simulink model "vhs_fpga_tx_10k_nosmq_nodsp"  (Simulink 7.1)
settings: Solver=ode45  StartTime=0.0  StopTime=inf  RelTol=1e-3
PreLoadFcn:
  | parameter();
undefined symbols (not defined in the file or in its folder): N1_CIC_PRESET1, N_FB_RX_frame, N_FB_TX_frame
libraries: xbsIndex_r4 x95, vhsadac_common_ob_fpgalib_v1_2_0 x10, misc_tools_dsplib_v1_0_0 x1, misc_tools_fpgalib_v1_0_0 x1, rffe_fpgalib_v1_1_0 x1, rtdex_fpgalib_v1_1_0 x1
(part 1 of 2)
settings Model: Creator=comlab  LastModifiedBy=lyrtech

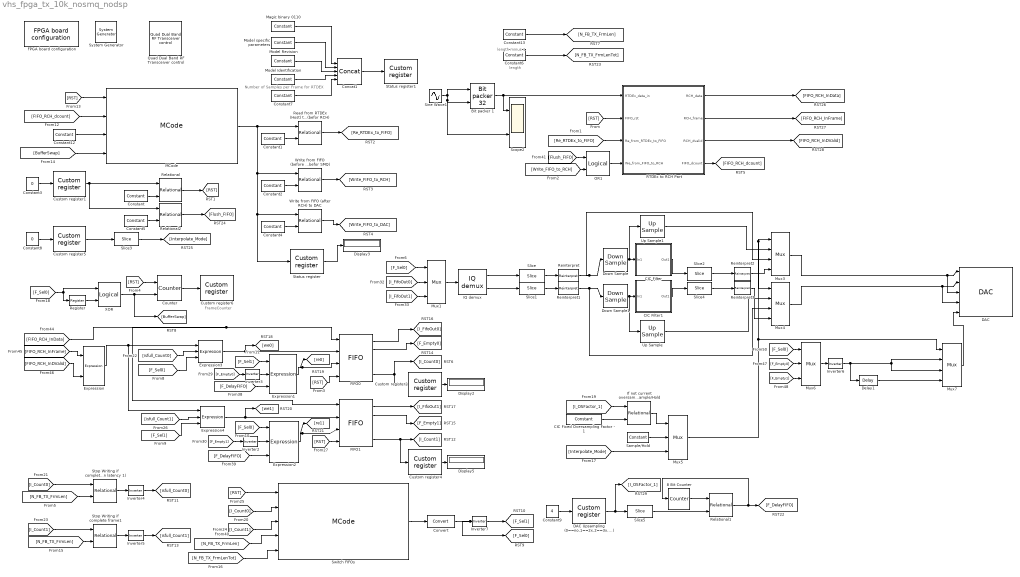
== system vhs_fpga_tx_10k_nosmq_nodsp ==
  note: FrameCounter
  note: length minus 1
  note: length
  note: Number of Samples per Frame for RTDEX
  " System Generator" : xbsIndex_r4/ System Generator  Tag=genX  SystemSampleTime=-1  xilinxfamily=virtex4  part=xc4vsx55  speed=-10  package=ff1148  synthesis_tool=XST  clock_wrapper=Clock Enables  directory=./netlist  testbench=off  simulink_period=1  sysclk_period=9  dcm_input_clock_period=100  incr_netlist=off  trim_vbits=Everywhere in SubSystem  dbl_ovrd=According to Block Masks  core_generation=According to Block Masks  run_coregen=off  deprecated_control=off  eval_field=0  block_type=sysgen
      settings: block_version=10.1.3
  8 Bit Counter : xbsIndex_r4/Counter  cnt_type=Free Running  cnt_to=Inf  operation=Up  start_count=0  cnt_by_val=1  arith_type=Unsigned  n_bits=8  bin_pt=0  load_pin=off  rst=on  en=off  explicit_period=on  period=1  dbl_ovrd=off  use_behavioral_HDL=off  use_rpm=off  implementation=Fabric  block_type=counter
      settings: block_version=VER_STRING_GOES_HERE
  Bit packer 1 : misc_tools_dsplib_v1_0_0/Bit packer 32  Tag=LYR_DSP_MISC_BIT_PACKER_32  Description=Lyrtech block  input_descriptor=[-16 -16]  data_type=double  frame_size=1
  CIC Filter : Subsystem  mask(CIC Filter){input_bitwidth=14, input_binpt=0, filter_type=Interpolator, rate_change=N1_CIC_PRESET1, stages=3, m=1, pipeline=on}
      mask prompts: input_bitwidth "Input Bit Width"; input_binpt "Input Binary Point"; filter_type "Filter Type"; rate_change "Sample Rate Change"; stages "Number of Stages"; m "Differential Delay"; pipeline "Pipeline Differentiators"
      mask help: Cascaded Integrated Comb (CIC) Filter
      mask init:
      | % CIC Single Channel v1.0
      | % Set Block Logo
      | sav_gcb=gcb;
      | [bg,fg] = xlcmap('XBlock',0);
      | iPos = get_param(sav_gcb,'Position');
      | iWidth=iPos(3)-iPos(1); iHeight=iPos(4)-iPos(2);
      | iCx=iWidth/2;
      | iCy=iHeight/2;
      | [logoX, logoY] = xlogo(iPos);
      | 
      | % Determine previous filter type and number of stages
      | prev_stages_list = find_system(sav_gcb, 'lookUnderMasks', 'all', 'FollowLinks', 'on', 'Regexp', 'on', 'Name', '^Integrator*'); %this is a cell array
      | prev_stages = length(prev_stages_list);
      | 
      | prev_filter_list = find_system(sav_gcb, 'lookUnderMasks', 'all', 'FollowLinks', 'on', 'Regexp', 'on', 'Name', '^Up Sample*'); %this is a cell array
      | if (isempty(prev_filter_list))
      |     prev_filter_list = find_system(sav_gcb, 'lookUnderMasks', 'all', 'FollowLinks', 'on', 'Regexp', 'on', 'Name', '^Down Sample*'); %this is a cell array
      |     if (isempty(prev_filter_list))
      |         errordlg('Previous Filter Type could not be determined')
      |     else
      |         prev_filter_type = 2;
      |     end
      | else
      |     prev_filter_type = 1;
      | end
      |   
      |   
      | % Print label on the block
      | if(filter_type == 2)
      |    cic_str = sprintf('%d-Stage\n CIC\n%d:1 Decimator',stages, rate_change);
      | else
      |    cic_str = sprintf('%d-Stage\n CIC\n1:%d Interpolator',stages, rate_change);	
      | end
      | 
      | % Make sure the entered values for stages and channels are positive integers
      | nstages = round(sum(abs(stages)));
      | 
      | % issue an error if the number of stages entered is zero
      | if (nstages == 0)
      | 	nstages = prev_stages;
      | 	errordlg('Number of Stages must be more than zero')
      | end
      | 
      | if (nstages == prev_stages) & (filter_type == prev_filter_type)
      |     return
      | end
      | 
      | if(filter_type == 2) % Decimator
      |    if (prev_filter_type == 1) % was interpolator so turn to decimator
      |        for i= 2:prev_stages,
      | 	      delete_line(sav_gcb, ['Integrator' int2str(i-1) '/' int2str(1)], ['Integrator' int2str(i) '/' int2str(1)]);
      | 	      delete_line(sav_gcb, ['Differentiator' int2str(i-1) '/' int2str(1)], ['Differentiator' int2str(i) '/' int2str(1)]);
      |        end
      | 
      |        % disconnect the last blocks in the two sections
      |        delete_line(sav_gcb, ['Differentiator' int2str(prev_stages) '/' int2str(1)], ['Up Sample/1']);
      |        delete_line(sav_gcb, ['Integrator' int2str(prev_stages) '/' int2str(1)], 'Out1/1');
      | 	
      | 	   % delete the line from the Up sampler to the Integrator
      | 	   delete_line(sav_gcb, 'Up Sample/1', 'Integrator1/1'); 
      | 	   delete_line(sav_gcb, 'In1/1', 'Differentiator1/1'); 
      | 	   
      | 	   % Delete the Up Sampler and then replace with an Down Sampler
      | 	   pup = get_param([sav_gcb '/Up Sample'], 'position');
      | 	   delete_block([sav_gcb '/Up Sample']);
      | 	   load_system('xbsIndex_r4');
      | 	   add_block('xbsIndex_r4/Down Sample', [sav_gcb '/Down Sample'], 'sample_ratio', 'rate_change','sample_phase', 'First Value of Frame', 'position', [pup(1), pup(2), pup(3),pup(4)]);
      | 	   
      | 	   % Switch the Integrators and Decimators around
      | 	   for i=1:prev_stages,
      | 		   tempi = get_param([sav_gcb '/Integrator' int2str(i)], 'position');
      | 	       tempd = get_param([sav_gcb '/Differentiator' int2str(i)], 'position');
      | 		   set_param([sav_gcb '/Differentiator' int2str(i)], 'position', [tempi(1), tempi(2), tempi(3), tempi(4)], 'output_bitwidth', 'ceil(stages*log2(rate_change*m) + input_bitwidth)');
      | 		   set_param([sav_gcb '/Integrator' int2str(i)], 'position', [tempd(1), tempd(2), tempd(3), tempd(4)]);
      | 	   end
      | 	   	   	
      | 	   % add back in the lines
      |        add_line(sav_gcb, 'In1/1', 'Integrator1/1', 'autorouting', 'on');
      | 	   add_line(sav_gcb, ['Integrator' int2str(prev_stages) '/1'], 'Down Sample/1', 'autorouting', 'on');
      | 	   add_line(sav_gcb, 'Down Sample/1', 'Differentiator1/1', 'autorouting', 'on');
      | 	   add_line(sav_gcb, ['Differentiator' int2str(prev_stages) '/1'], 'Out1/1', 'autorouting', 'on');
      | 	   for i= 2:prev_stages,
      |           add_line(sav_gcb, ['Integrator' int2str(i-1) '/1'], ['Integrator' int2str(i) '/' int2str(1)], 'autorouting', 'on');
      |           add_line(sav_gcb, ['Differentiator' int2str(i-1) '/1'], ['Differentiator' int2str(i) '/' int2str(1)], 'autorouting', 'on');
      | 	   end
      | 		
      |        %Set the Output bit widths of Differentiator and Integrator stages
      |        set_param([sav_gcb '/Differentiator1'], 'output_bitwidth', 'ceil(stages*log2(rate_change*m) + input_bitwidth)');
      | 	   	   %Set the Output bit width of Integrator stages
      | 	   %Calculate the Interpolator Integrator Output Bit Growth
      |        for i= 1:prev_stages,
      | 			 j = nstages+i;
      | 	         set_param([sav_gcb '/Integrator' int2str(i)], 'output_bitwidth', 'ceil(stages*log2(rate_change*m) + input_bitwidth)');
      |              set_param([sav_gcb '/Differentiator' int2str(i)], 'output_bitwidth', 'ceil(stages*log2(rate_change*m) + input_bitwidth)');
      | 	   end
      | 	   
      |    end
      |    
      |    if (nstages ~= prev_stages)
      |     
      |        % disconnect all the wires from all the blocks
      |        for i= 2:prev_stages,
      | 	      delete_line(sav_gcb, ['Integrator' int2str(i-1) '/' int2str(1)], ['Integrator' int2str(i) '/' int2str(1)]);
      | 	      delete_line(sav_gcb, ['Differentiator' int2str(i-1) '/' int2str(1)], ['Differentiator' int2str(i) '/' int2str(1)]);
      |        end
      | 
      |        % disconnect the last blocks in the two sections
      |        delete_line(sav_gcb, ['Integrator' int2str(prev_stages) '/' int2str(1)], ['Down Sample/1']);
      |        delete_line(sav_gcb, ['Differentiator' int2str(prev_stages) '/' int2str(1)], 'Out1/1');
      | 	
      | 	   % delete the line from the down sampler to the differentiator
      | 	   delete_line(sav_gcb, 'Down Sample/1', 'Differentiator1/1');
      | 	
      | 	   % Remove all the blocks except the first one (as we always will have one)
      |        for i=2:prev_stages,
      | 		  delete_block([sav_gcb '/Differentiator' int2str(i)]);
      | 	      delete_block([sav_gcb '/Integrator' int2str(i)]);
      |        end
      | 	   
      | 	   %Set the Output bit width of Differentiator stages
      |        set_param([sav_gcb '/Differentiator1'], 'output_bitwidth', 'ceil(stages*log2(rate_change*m) + input_bitwidth)');
      | 	   
      | 	   % collect data on the position of existing blocks
      | 	   pi = get_param([sav_gcb '/Integrator1'], 'position');
      | 	   pd = get_param([sav_gcb '/Differentiator1'], 'position');
      | 	   set_param([sav_gcb '/Differentiator1'], 'position', [pi(1)+(nstages+1)*80, pd(2), pi(3)+(nstages+1)*80, pd(4)]);
      | 	   pd = get_param([sav_gcb '/Differentiator1'], 'position');
      | 	
      | 	   % move the current blocks to accomadate for new blocks to be added 
      | 	   pds = get_param([sav_gcb '/Down Sample'], 'position');
      | 	   set_param([sav_gcb '/Down Sample'], 'position', [pi(1)+(nstages)*80, pds(2), pi(3)+(nstages)*80, pds(4)]);
      | 	   
      | 	   po = get_param([sav_gcb '/Out1'], 'position');
      | 	   set_param([sav_gcb '/Out1'], 'position', [pd(1)+(nstages+1)*80, po(2), pd(1)+(po(3)-po(1))+(nstages+1)*80, po(4)]);	
      | 	
      | 	   % add back in the line between the Down Sampler and the 1st Differentiator
      |        add_line(sav_gcb, 'Down Sample/1', ['Differentiator1/' int2str(1)], 'autorouting', 'on');
      | 
      | 	   % Only add blocks if more than one stage is required
      | 	   if (nstages ~= 1)
      | 		
      | 	       % Add in a copy of the first block to make up the required number of stages
      |            for i=2:nstages,
      |                add_block([sav_gcb '/Integrator1'], [sav_gcb '/Integrator' int2str(i)], 'position', [pi(1)+(i-1)*80, pi(2), pi(3)+(i-1)*80, pi(4)]);
      | 		       add_block([sav_gcb '/Differentiator1'], [sav_gcb '/Differentiator' int2str(i)], 'position', [pd(1)+(i-1)*80, pd(2), pd(3)+(i-1)*80, pd(4)]);
      | 	       end
      | 		
      | 	       % Connect up the wires to each block use autorouting
      |            for i= 2:nstages,
      |  		       add_line(sav_gcb, ['Integrator' int2str(i-1) '/' int2str(1)], ['Integrator' int2str(i) '/' int2str(1)], 'autorouting', 'on');
      | 	           add_line(sav_gcb, ['Differentiator' int2str(i-1) '/' int2str(1)], ['Differentiator' int2str(i) '/' int2str(1)], 'autorouting', 'on');
      |            end
      | 	    end
      | 	       % Connect the last blocks in the two sections
      |            add_line(sav_gcb, ['Integrator' int2str(nstages) '/' int2str(1)], ['Down Sample/1'], 'autorouting', 'on');
      |            add_line(sav_gcb, ['Differentiator' int2str(nstages) '/' int2str(1)], ['Out1/1'], 'autorouting', 'on');
      |    end
      | 
      | else % Interpolator
      |    
      | 	
      | 	if (prev_filter_type == 2) % was decimator so turn to interpolator
      | 	
      | 	  % disconnect all the wires from all the blocks
      |        for i= 2:prev_stages,
      | 	      delete_line(sav_gcb, ['Integrator' int2str(i-1) '/' int2str(1)], ['Integrator' int2str(i) '/' int2str(1)]);
      | 	      delete_line(sav_gcb, ['Differentiator' int2str(i-1) '/' int2str(1)], ['Differentiator' int2str(i) '/' int2str(1)]);
      |        end
      | 
      |        % disconnect the last blocks in the two sections
      |        delete_line(sav_gcb, ['Integrator' int2str(prev_stages) '/' int2str(1)], ['Down Sample/1']);
      |        delete_line(sav_gcb, ['Differentiator' int2str(prev_stages) '/' int2str(1)], 'Out1/1');
      | 	
      | 	   % delete the line from the down sampler to the Differentiator
      | 	   delete_line(sav_gcb, 'Down Sample/1', 'Differentiator1/1'); 
      | 	   delete_line(sav_gcb, 'In1/1', 'Integrator1/1'); 
      | 	   
      | 	   % Delete the Down Sampler and then replace with a Up Sampler
      | 	   pdwn = get_param([sav_gcb '/Down Sample'], 'position');
      | 	   delete_block([sav_gcb '/Down Sample']);
      | 	   load_system('xbsIndex_r4');
      | 	   add_block('xbsIndex_r4/Up Sample', [sav_gcb '/Up Sample'], 'sample_ratio', 'rate_change', 'position', [pdwn(1), pdwn(2), pdwn(3), pdwn(4)]);
      | 	   
      | 	   % Switch the Integrators and Decimators around
      | 	   for i=1:prev_stages,
      | 		   tempi = get_param([sav_gcb '/Integrator' int2str(i)], 'position');
      | 	       tempd = get_param([sav_gcb '/Differentiator' int2str(i)], 'position');
      | 		   set_param([sav_gcb '/Differentiator' int2str(i)], 'position', [tempi(1), tempi(2), tempi(3), tempi(4)], 'output_bitwidth', [int2str(i) '+ input_bitwidth']);
      | 		   set_param([sav_gcb '/Integrator' int2str(i)], 'position', [tempd(1), tempd(2), tempd(3), tempd(4)]);
      | 	   end
      | 	   	   	
      | 	   % add back in the lines
      |        add_line(sav_gcb, 'In1/1', 'Differentiator1/1', 'autorouting', 'on');
      | 	   add_line(sav_gcb, ['Differentiator' int2str(prev_stages) '/1'], 'Up Sample/1', 'autorouting', 'on');
      | 	   add_line(sav_gcb, 'Up Sample/1', 'Integrator1/1', 'autorouting', 'on');
      | 	   add_line(sav_gcb, ['Integrator' int2str(prev_stages) '/1'], 'Out1/1', 'autorouting', 'on');
      | 	   for i= 2:prev_stages,
      |           add_line(sav_gcb, ['Integrator' int2str(i-1) '/1'], ['Integrator' int2str(i) '/1'], 'autorouting', 'on');
      |           add_line(sav_gcb, ['Differentiator' int2str(i-1) '/1'], ['Differentiator' int2str(i) '/1'], 'autorouting', 'on');
      | 	   end
      | 	   
      | 	   %Set the Output bit width of Integrator stages
      | 	   %Calculate the Interpolator Integrator Output Bit Growth
      |        for i= 1:prev_stages,
      | 			 j = nstages+i;
      | 	         set_param([sav_gcb '/Integrator' int2str(i)], 'output_bitwidth', ['ceil(log2(2^(2*stages-' int2str(j) ')*(rate_change*m)^(' int2str(j) '-stages)) + input_bitwidth)']);
      | 	   end
      | 		
      |    end
      |    
      | 	
      | 	if (nstages ~= prev_stages)
      |     
      |        % disconnect all the wires from all the blocks
      |        for i= 2:prev_stages,
      | 	      delete_line(sav_gcb, ['Integrator' int2str(i-1) '/' int2str(1)], ['Integrator' int2str(i) '/' int2str(1)]);
      | 	      delete_line(sav_gcb, ['Differentiator' int2str(i-1) '/' int2str(1)], ['Differentiator' int2str(i) '/' int2str(1)]);
      |        end
      | 
      |        % disconnect the last blocks in the two sections
      |        delete_line(sav_gcb, ['Differentiator' int2str(prev_stages) '/' int2str(1)], ['Up Sample/1']);
      |        delete_line(sav_gcb, ['Integrator' int2str(prev_stages) '/' int2str(1)], 'Out1/1');
      |        
      | 	
      | 	   % delete the line from the Up sampler to the Integrator1 for movement later
      | 	   delete_line(sav_gcb, 'Up Sample/1', 'Integrator1/1'); 
      | 	
      | 	   % Remove all the blocks except the first one (as we always will have one)
      |        for i=2:prev_stages,
      | 		  delete_block([sav_gcb '/Differentiator' int2str(i)]);
      | 	      delete_block([sav_gcb '/Integrator' int2str(i)]);
      |        end
      | 	
      | 	   %Set the Output bit width of first Differentiator stage (other are set as copies of this block)
      |        set_param([sav_gcb '/Differentiator1'], 'output_bitwidth', '1 + input_bitwidth');
      | 	   
      | 	   % collect data on the position of existing blocks
      | 	   pi = get_param([sav_gcb '/Integrator1'], 'position');
      | 	   pd = get_param([sav_gcb '/Differentiator1'], 'position');
      | 	   set_param([sav_gcb '/Integrator1'], 'position', [pd(1)+(nstages+1)*80, pi(2), pd(3)+(nstages+1)*80, pi(4)]);
      | 	   pi = get_param([sav_gcb '/Integrator1'], 'position');
      | 	
      | 	   % move the current blocks to accomadate for new blocks to be added 
      | 	   pus = get_param([sav_gcb '/Up Sample'], 'position');
      | 	   set_param([sav_gcb '/Up Sample'], 'position', [pd(1)+(nstages)*80, pus(2), pd(3)+(nstages)*80, pus(4)]);
      | 	
      | 	   po = get_param([sav_gcb '/Out1'], 'position');
      |        set_param([sav_gcb '/Out1'], 'position', [pi(1)+(nstages+1)*80, po(2), pi(1)+(po(3)-po(1))+(nstages+1)*80, po(4)]);	
      |       
      | 	
      | 	   % add back in the line between the Up Sampler and the 1st Integrator1
      | 	   add_line(sav_gcb, 'Up Sample/1', 'Integrator1/1', 'autorouting', 'on');
      | 	   
      | 	   % Only add blocks if more than one stage is required
      | 	   if (nstages ~= 1)
      | 		
      | 	       % Add in a copy of the first block to make up the required number of stages
      |            for i=2:nstages,
      |                add_block([sav_gcb '/Integrator1'], [sav_gcb '/Integrator' int2str(i)], 'position', [pi(1)+(i-1)*80, pi(2), pi(3)+(i-1)*80, pi(4)]);
      | 		       add_block([sav_gcb '/Differentiator1'], [sav_gcb '/Differentiator' int2str(i)], 'position', [pd(1)+(i-1)*80, pd(2), pd(3)+(i-1)*80, pd(4)], 'output_bitwidth', [int2str(i) '+ input_bitwidth']);
      | 	       end
      | 		
      | 	       % Connect up the wires to each block use autorouting
      |            for i= 2:nstages,
      |  		       add_line(sav_gcb, ['Integrator' int2str(i-1) '/' int2str(1)], ['Integrator' int2str(i) '/' int2str(1)], 'autorouting', 'on');
      | 	           add_line(sav_gcb, ['Differentiator' int2str(i-1) '/' int2str(1)], ['Differentiator' int2str(i) '/' int2str(1)], 'autorouting', 'on');
      |            end
      | 	    end
      | 	       % Connect the last blocks in the two sections
      |            add_line(sav_gcb, ['Differentiator' int2str(nstages) '/1'], ['Up Sample/1'], 'autorouting', 'on');
      |            add_line(sav_gcb, ['Integrator' int2str(nstages) '/1'], ['Out1/1'], 'autorouting', 'on');
      | 		   
      | 	     %Set the Output bit width of Integrator stages
      | 	     %Calculate the Interpolator Integrator Output Bit Growth
      |           for i= 1:nstages,
      | 			 j = nstages+i;
      | 	         set_param([sav_gcb '/Integrator' int2str(i)], 'output_bitwidth', ['ceil(log2(2^(2*stages-' int2str(j) ')*(rate_change*m)^(' int2str(j) '-stages)) + input_bitwidth)']);
      | 	      end
      |    end
      | 	  
      | end
      | 
      | 
      | % Set the pipelining to ON or OFF on the differentiators
      | if (pipeline == 0)
      | 	for i= 1:nstages
      | 		set_param([sav_gcb '/Differentiator' int2str(i), '/AddSub'], 'latency', '0')
      | 	end
      | else
      | 	for i= 1:nstages
      | 		set_param([sav_gcb '/Differentiator' int2str(i), '/AddSub'], 'latency' ,'1')
      | 	end
      | end
      settings: CopyFcn=set_param(gcb, 'MaskSelfModifiable', 'on', 'LinkStatus', 'none');
      mask Help: eval('');xlDoc('-book','sysgen','-topic','CIC_Filter');
      mask StyleString: edit,edit,popup(Interpolator|Decimator),edit,edit,popup(1|2|3|4),checkbox
      mask Display:
      | patch([0 iWidth iWidth 0],[0 0 iHeight iHeight] , bg);
      | patch(logoX,logoY , fg);
      | plot([0 0 iWidth iWidth 0], [0 iHeight iHeight 0 0]);
      | disp(cic_str)
  CIC Filter1 : Subsystem  mask(CIC Filter){input_bitwidth=14, input_binpt=0, filter_type=Interpolator, rate_change=N1_CIC_PRESET1, stages=3, m=1, pipeline=on}
      mask prompts: input_bitwidth "Input Bit Width"; input_binpt "Input Binary Point"; filter_type "Filter Type"; rate_change "Sample Rate Change"; stages "Number of Stages"; m "Differential Delay"; pipeline "Pipeline Differentiators"
      mask help: Cascaded Integrated Comb (CIC) Filter
      mask init: same as vhs_fpga_tx_10k_nosmq_nodsp/CIC Filter
      settings: CopyFcn=set_param(gcb, 'MaskSelfModifiable', 'on', 'LinkStatus', 'none');
      mask Help: eval('');xlDoc('-book','sysgen','-topic','CIC_Filter');
      mask StyleString: edit,edit,popup(Interpolator|Decimator),edit,edit,popup(1|2|3|4),checkbox
      mask Display:
      | patch([0 iWidth iWidth 0],[0 0 iHeight iHeight] , bg);
      | patch(logoX,logoY , fg);
      | plot([0 0 iWidth iWidth 0], [0 iHeight iHeight 0 0]);
      | disp(cic_str)
  CIC Fixed Oversampling Factor - 1 : xbsIndex_r4/Constant  arith_type=Unsigned  const=N1_CIC_PRESET1-1  n_bits=32  bin_pt=0  explicit_period=on  period=1  equ=P=C  opselect=C  inp2=PCIN>>17  opr=+  inp1=P  carry=CIN  dbl_ovrd=off  block_type=constant
  Concat1 : xbsIndex_r4/Concat  num_inputs=5  dbl_ovrd=off  block_type=concat
      settings: block_version=10.1.3
  Constant : xbsIndex_r4/Constant  arith_type=Unsigned  const=1  n_bits=32  bin_pt=0  explicit_period=off  period=1  equ=P=C  opselect=C  inp2=PCIN>>17  opr=+  inp1=P  carry=CIN  dbl_ovrd=off  block_type=constant
  Constant1 : xbsIndex_r4/Constant  arith_type=Unsigned  const=1  n_bits=32  bin_pt=0  explicit_period=on  period=1  equ=P=C  opselect=C  inp2=PCIN>>17  opr=+  inp1=P  carry=CIN  dbl_ovrd=off  block_type=constant
  Constant12 : xbsIndex_r4/Constant  arith_type=Unsigned  const=N_FB_RX_frame  n_bits=14  bin_pt=0  explicit_period=on  period=1  equ=P=C  opselect=C  inp2=PCIN>>17  opr=+  inp1=P  carry=CIN  dbl_ovrd=off  block_type=constant
  Constant13 : xbsIndex_r4/Constant  arith_type=Unsigned  const=N_FB_TX_frame-1  n_bits=14  bin_pt=0  explicit_period=on  period=1  equ=P=C  opselect=C  inp2=PCIN>>17  opr=+  inp1=P  carry=CIN  dbl_ovrd=off  block_type=constant
  Constant2 : xbsIndex_r4/Constant  arith_type=Unsigned  const=2  n_bits=32  bin_pt=0  explicit_period=on  period=1  equ=P=C  opselect=C  inp2=PCIN>>17  opr=+  inp1=P  carry=CIN  dbl_ovrd=off  block_type=constant
  Constant3 : Constant  Value=0  OutDataType=sfix(16)  OutScaling=2^0  SampleTime=1
  Constant4 : xbsIndex_r4/Constant  arith_type=Unsigned  const=3  n_bits=32  bin_pt=0  explicit_period=on  period=1  equ=P=C  opselect=C  inp2=PCIN>>17  opr=+  inp1=P  carry=CIN  dbl_ovrd=off  block_type=constant
  Constant5 : xbsIndex_r4/Constant  arith_type=Unsigned  const=2  n_bits=32  bin_pt=0  explicit_period=off  period=1  equ=P=C  opselect=C  inp2=PCIN>>17  opr=+  inp1=P  carry=CIN  dbl_ovrd=off  block_type=constant
  Constant6 : xbsIndex_r4/Constant  arith_type=Unsigned  const=N_FB_TX_frame  n_bits=14  bin_pt=0  explicit_period=on  period=1  equ=P=C  opselect=C  inp2=PCIN>>17  opr=+  inp1=P  carry=CIN  dbl_ovrd=off  block_type=constant
  Constant7 : xbsIndex_r4/Constant  arith_type=Unsigned  const=N_FB_RX_frame  n_bits=15  bin_pt=0  explicit_period=on  period=1  equ=P=C  opselect=C  inp2=PCIN>>17  opr=+  inp1=P  carry=CIN  dbl_ovrd=off  block_type=constant
  Constant8 : Constant  Value=0  OutDataType=sfix(16)  OutScaling=2^0  SampleTime=1
  Constant9 : Constant  Value=4  OutDataType=sfix(16)  OutScaling=2^0  SampleTime=1
  Convert : xbsIndex_r4/Convert  arith_type=Boolean  n_bits=1  bin_pt=0  quantization=Truncate  overflow=Wrap  latency=2  dbl_ovrd=off  pipeline=off  block_type=convert
      settings: block_version=10.1.3
  Counter : xbsIndex_r4/Counter  cnt_type=Free Running  cnt_to=Inf  operation=Up  start_count=0  cnt_by_val=1  arith_type=Unsigned  n_bits=32  bin_pt=0  load_pin=off  rst=on  en=on  explicit_period=on  period=1  dbl_ovrd=off  use_behavioral_HDL=off  use_rpm=off  implementation=Fabric  block_type=counter
  Custom register1 : vhsadac_common_ob_fpgalib_v1_2_0/Custom register  Tag=LYR_FPGA_IO_CUSTOM_REGISTER  Description=Lyrtech block  SystemSampleTime=-1  regID=1  direction=Read  output_arithmetic_type=Unsigned  output_width=32  binpt=0  sample_period=1
  Custom register2 : vhsadac_common_ob_fpgalib_v1_2_0/Custom register  Tag=LYR_FPGA_IO_CUSTOM_REGISTER  Description=Lyrtech block  SystemSampleTime=-1  regID=3  direction=Write  output_arithmetic_type=Unsigned  output_width=32  binpt=0  sample_period=1
  Custom register4 : vhsadac_common_ob_fpgalib_v1_2_0/Custom register  Tag=LYR_FPGA_IO_CUSTOM_REGISTER  Description=Lyrtech block  SystemSampleTime=-1  regID=4  direction=Write  output_arithmetic_type=Unsigned  output_width=32  binpt=0  sample_period=1
  Custom register5 : vhsadac_common_ob_fpgalib_v1_2_0/Custom register  Tag=LYR_FPGA_IO_CUSTOM_REGISTER  Description=Lyrtech block  SystemSampleTime=-1  regID=2  direction=Read  output_arithmetic_type=Unsigned  output_width=32  binpt=0  sample_period=1
  Custom register6 : vhsadac_common_ob_fpgalib_v1_2_0/Custom register  Tag=LYR_FPGA_IO_CUSTOM_REGISTER  Description=Lyrtech block  SystemSampleTime=-1  regID=6  direction=Write  output_arithmetic_type=Unsigned  output_width=32  binpt=0  sample_period=1
  DAC : vhsadac_common_ob_fpgalib_v1_2_0/DAC  Tag=LYR_FPGA_IO_DAC  Description=Lyrtech block  SystemSampleTime=-1  nbofcha=4  binpt=0  sample_period=1  trig_sig=off  run_sig=on
  "DAC Upsampling (0==no,1==2x,2==3x,...) " : vhsadac_common_ob_fpgalib_v1_2_0/Custom register  Tag=LYR_FPGA_IO_CUSTOM_REGISTER  Description=Lyrtech block  SystemSampleTime=-1  regID=5  direction=Read  output_arithmetic_type=Unsigned  output_width=32  binpt=0  sample_period=1
  Delay1 : xbsIndex_r4/Delay  en=off  latency=30-5  dbl_ovrd=off  reg_retiming=off  block_type=delay
  Display2 : Display
  Display3 : Display
  Display5 : Display
  Down Sample : xbsIndex_r4/Down Sample  sample_ratio=N1_CIC_PRESET1  sample_phase="Last Value of Frame  (most efficient)"  en=off  latency=1  dbl_ovrd=off  block_type=dsamp
      settings: block_version=10.1.3
  Down Sample1 : xbsIndex_r4/Down Sample  sample_ratio=N1_CIC_PRESET1  sample_phase="Last Value of Frame  (most efficient)"  en=off  latency=1  dbl_ovrd=off  block_type=dsamp
      settings: block_version=10.1.3
  Expression : xbsIndex_r4/Expression  expression=a & b  align_bp=on  en=off  latency=0  precision=Full  arith_type=Unsigned  n_bits=16  bin_pt=0  dbl_ovrd=off  block_type=expr
      settings: block_version=10.1.3
  Expression{1..4} (4 alike) : xbsIndex_r4/Expression  expression=a & b & c  align_bp=on  en=off  latency=0  precision=Full  arith_type=Unsigned  n_bits=16  bin_pt=0  dbl_ovrd=off  block_type=expr
      settings: block_version=10.1.3
  FIFO0 : xbsIndex_r4/FIFO  depth=16K  percent_nbits=1  rst=on  en=off  use_dcount=on  use_almost_empty=off  almost_empty_thresh=2  use_almost_full=off  almost_full_thresh=14  dbl_ovrd=off  mem_type=Block RAM  block_type=fifo
      settings: block_version=10.1.3
  FIFO1 : xbsIndex_r4/FIFO  depth=16K  percent_nbits=1  rst=on  en=off  use_dcount=on  use_almost_empty=off  almost_empty_thresh=2  use_almost_full=off  almost_full_thresh=14  dbl_ovrd=off  mem_type=Block RAM  block_type=fifo
      settings: block_version=10.1.3
  FPGA board configuration : vhsadac_common_ob_fpgalib_v1_2_0/FPGA board configuration  Tag=SysgenCompile  Description=Lyrtech block  SystemSampleTime=-1  clk_sel=Hardware implementation  clk_src=ADC/DAC clock  hardware=VHS-DAC Virtex-4  copy_bit_cd=on
  IQ demux : misc_tools_fpgalib_v1_0_0/IQ demux  Tag=LYR_FPGA_MISC_IQ_DEMUX  Description=Lyrtech block  SystemSampleTime=-1
  "If not current oversampling factor is not fixed CIC oversampling, ignore Interpolate mode and do  Sample/Hold" : xbsIndex_r4/Relational  mode=a=b  en=off  latency=0  dbl_ovrd=off  block_type=relational
      settings: block_version=10.1.3
  Inverter2 : xbsIndex_r4/Inverter  en=off  latency=0  dbl_ovrd=off  block_type=inv
  Inverter3 : xbsIndex_r4/Inverter  en=off  latency=0  dbl_ovrd=off  block_type=inv
  Inverter4 : xbsIndex_r4/Inverter  en=off  latency=1  dbl_ovrd=off  block_type=inv
  Inverter5 : xbsIndex_r4/Inverter  en=off  latency=1  dbl_ovrd=off  block_type=inv
  Inverter6 : xbsIndex_r4/Inverter  en=off  latency=5  dbl_ovrd=off  block_type=inv
  Inverter7 : xbsIndex_r4/Inverter  en=off  latency=0  dbl_ovrd=off  block_type=inv
  MCode : xbsIndex_r4/MCode  mfname=state_machine_tx  explicit_period=off  period=1  inputsTable={'boundInpExpr'=>['','','',''],'inputs'=>['RST','FIFO_RCH_dcount','N_FB_RX_frame','F_BufferSwap']}  outputsTable={'outputs'=>['sel'],'suppressOut'=>['off']}  dbl_ovrd=off  enable_stdout=off  enable_debug=off  suppress_output=1  defparams={}  hide_port_list={}  block_type=mcode
      settings: block_version=10.1.3
  Magic binary 0110 : xbsIndex_r4/Constant  arith_type=Unsigned  const=6  n_bits=4  bin_pt=0  explicit_period=on  period=1  equ=P=C  opselect=C  inp2=PCIN>>17  opr=+  inp1=P  carry=CIN  dbl_ovrd=off  block_type=constant
  Model Identification : xbsIndex_r4/Constant  arith_type=Unsigned  const=3  n_bits=4  bin_pt=0  explicit_period=on  period=1  equ=P=C  opselect=C  inp2=PCIN>>17  opr=+  inp1=P  carry=CIN  dbl_ovrd=off  block_type=constant
  Model Revision : xbsIndex_r4/Constant  arith_type=Unsigned  const=2  n_bits=3  bin_pt=0  explicit_period=on  period=1  equ=P=C  opselect=C  inp2=PCIN>>17  opr=+  inp1=P  carry=CIN  dbl_ovrd=off  block_type=constant
  Model specific parameters : xbsIndex_r4/Constant  arith_type=Unsigned  const=0  n_bits=6  bin_pt=0  explicit_period=on  period=1  equ=P=C  opselect=C  inp2=PCIN>>17  opr=+  inp1=P  carry=CIN  dbl_ovrd=off  block_type=constant
  Mux1 : xbsIndex_r4/Mux  inputs=2  en=off  latency=0  precision=Full  arith_type=Unsigned  n_bits=16  bin_pt=14  quantization=Truncate  overflow=Wrap  dbl_ovrd=off  block_type=mux
  Mux3 : xbsIndex_r4/Mux  inputs=3  en=off  latency=0  precision=Full  arith_type=Unsigned  n_bits=16  bin_pt=14  quantization=Truncate  overflow=Wrap  dbl_ovrd=off  block_type=mux
  Mux4 : xbsIndex_r4/Mux  inputs=3  en=off  latency=0  precision=Full  arith_type=Unsigned  n_bits=16  bin_pt=14  quantization=Truncate  overflow=Wrap  dbl_ovrd=off  block_type=mux
  Mux5 : xbsIndex_r4/Mux  inputs=2  en=off  latency=0  precision=Full  arith_type=Unsigned  n_bits=16  bin_pt=14  quantization=Truncate  overflow=Wrap  dbl_ovrd=off  block_type=mux
  Mux6 : xbsIndex_r4/Mux  inputs=2  en=off  latency=0  precision=Full  arith_type=Unsigned  n_bits=16  bin_pt=14  quantization=Truncate  overflow=Wrap  dbl_ovrd=off  block_type=mux
  Mux7 : xbsIndex_r4/Mux  inputs=3  en=off  latency=0  precision=Full  arith_type=Unsigned  n_bits=16  bin_pt=14  quantization=Truncate  overflow=Wrap  dbl_ovrd=off  block_type=mux
  OR1 : xbsIndex_r4/Logical  logical_function=OR  inputs=2  en=off  latency=0  precision=Full  arith_type=Unsigned  n_bits=16  bin_pt=0  align_bp=on  dbl_ovrd=off  block_type=logical
  Quad Dual Band RF Transceiver control : rffe_fpgalib_v1_1_0/Quad Dual Band RF Transceiver control  Tag=LYR_FPGA_CONTROL_QUAD_DUAL_BAND_RF_TRANSCEIVER_CONTROL  Description=Lyrtech block  SystemSampleTime=-1  external_gain=off  tx1=off  tx2=off  tx3=off  tx4=off  mode=off  add=off  int_divider=off  frac_divider=off  int_divider_en=off  frac_divider_en=off  lock_detect=off  sample_period=1
  RTDEx to RCH Part : Subsystem
  Read from RTDEx (Host) to FIFO (befor RCH) : xbsIndex_r4/Relational  mode=a=b  en=off  latency=1  dbl_ovrd=off  block_type=relational
      settings: block_version=10.1.3
  Register : xbsIndex_r4/Register  init=0  rst=off  en=off  dbl_ovrd=off  block_type=register
  Reinterpret{,1..3} (4 alike) : xbsIndex_r4/Reinterpret  force_arith_type=on  arith_type="Signed  (2's comp)"  force_bin_pt=on  bin_pt=0  block_type=reinterpret
      settings: infoedit="Changes signal type without altering the binary representation.   You can changed the signal between signed and unsigned, and relocate the binary point.<P><P>Hardware notes: In hardware this block costs nothing.<P><P>Example:  Suppose the input is 6 bits wide, signed, with 2 fractional bits, and the output is forced to unsigned with 0 fractional bits.  Then an input of -2.0 (1110.00 in binary 2's complement) becomes an output of 56 (111000 in binary)."  block_version=10.1.3
  Relational : xbsIndex_r4/Relational  mode=a=b  en=off  latency=1  dbl_ovrd=off  block_type=relational
      settings: block_version=10.1.3
  Relational1 : xbsIndex_r4/Relational  mode=a=b  en=off  latency=0  dbl_ovrd=off  block_type=relational
      settings: block_version=VER_STRING_GOES_HERE
  Relational2 : xbsIndex_r4/Relational  mode=a=b  en=off  latency=1  dbl_ovrd=off  block_type=relational
      settings: block_version=10.1.3
  Sample/Hold : xbsIndex_r4/Constant  arith_type=Unsigned  const=1  n_bits=2  bin_pt=0  explicit_period=on  period=1  equ=P=C  opselect=C  inp2=PCIN>>17  opr=+  inp1=P  carry=CIN  dbl_ovrd=off  block_type=constant
  Scope2 : Scope  NumInputPorts=2
      settings: YMin=-5~-5  YMax=5~5  MaxDataPoints=500000
  Sine Wave1 : Sin  SineType=Sample based  Amplitude=2^13  Samples=50  SampleTime=1
  Slice : xbsIndex_r4/Slice  nbits=14  boolean_output=off  mode=Upper Bit Location + Width  bit1=0  base1=MSB of Input  bit0=0  base0=LSB of Input  dbl_ovrd=off  block_type=slice
      settings: infoedit="Extracts a given range of bits from each input sample and presents it at the output.  The output type is ordinarily unsigned with binary point at zero, but can be Boolean when the slice is one bit wide.<P><P>Hardware notes: In hardware this block costs nothing."  block_version=10.1.3
  Slice1 : xbsIndex_r4/Slice  nbits=14  boolean_output=off  mode=Upper Bit Location + Width  bit1=0  base1=MSB of Input  bit0=0  base0=LSB of Input  dbl_ovrd=off  block_type=slice
      settings: infoedit="Extracts a given range of bits from each input sample and presents it at the output.  The output type is ordinarily unsigned with binary point at zero, but can be Boolean when the slice is one bit wide.<P><P>Hardware notes: In hardware this block costs nothing."  block_version=10.1.3
  Slice2 : xbsIndex_r4/Slice  nbits=14  boolean_output=off  mode=Upper Bit Location + Width  bit1=-2  base1=MSB of Input  bit0=0  base0=LSB of Input  dbl_ovrd=off  block_type=slice
      settings: infoedit="Extracts a given range of bits from each input sample and presents it at the output.  The output type is ordinarily unsigned with binary point at zero, but can be Boolean when the slice is one bit wide.<P><P>Hardware notes: In hardware this block costs nothing."  block_version=10.1.3
  Slice3 : xbsIndex_r4/Slice  nbits=2  boolean_output=off  mode=Lower Bit Location + Width  bit1=0  base1=MSB of Input  bit0=0  base0=LSB of Input  dbl_ovrd=off  block_type=slice
      settings: infoedit="Extracts a given range of bits from each input sample and presents it at the output.  The output type is ordinarily unsigned with binary point at zero, but can be Boolean when the slice is one bit wide.<P><P>Hardware notes: In hardware this block costs nothing."  block_version=10.1.3
  Slice4 : xbsIndex_r4/Slice  nbits=14  boolean_output=off  mode=Upper Bit Location + Width  bit1=-2  base1=MSB of Input  bit0=0  base0=LSB of Input  dbl_ovrd=off  block_type=slice
      settings: infoedit="Extracts a given range of bits from each input sample and presents it at the output.  The output type is ordinarily unsigned with binary point at zero, but can be Boolean when the slice is one bit wide.<P><P>Hardware notes: In hardware this block costs nothing."  block_version=10.1.3
  Slice5 : xbsIndex_r4/Slice  nbits=8  boolean_output=off  mode=Lower Bit Location + Width  bit1=-4  base1=MSB of Input  bit0=0  base0=LSB of Input  dbl_ovrd=off  block_type=slice
      settings: infoedit="Extracts a given range of bits from each input sample and presents it at the output.  The output type is ordinarily unsigned with binary point at zero, but can be Boolean when the slice is one bit wide.<P><P>Hardware notes: In hardware this block costs nothing."  block_version=10.1.3
  Status register : vhsadac_common_ob_fpgalib_v1_2_0/Custom register  Tag=LYR_FPGA_IO_CUSTOM_REGISTER  Description=Lyrtech block  SystemSampleTime=-1  regID=0  direction=Write  output_arithmetic_type=Unsigned  output_width=32  binpt=0  sample_period=1
  Status register1 : vhsadac_common_ob_fpgalib_v1_2_0/Custom register  Tag=LYR_FPGA_IO_CUSTOM_REGISTER  Description=Lyrtech block  SystemSampleTime=-1  regID=7  direction=Write  output_arithmetic_type=Unsigned  output_width=32  binpt=0  sample_period=1
  "Stop Writing if complete frame (tests for len-1, then latency 1)" : xbsIndex_r4/Relational  mode=a=b  en=off  latency=0  dbl_ovrd=off  block_type=relational
      settings: block_version=10.1.3
  Stop Writing if complete frame1 : xbsIndex_r4/Relational  mode=a=b  en=off  latency=0  dbl_ovrd=off  block_type=relational
      settings: block_version=10.1.3
  Switch FIFOs : xbsIndex_r4/MCode  mfname=state_machine_fifos  explicit_period=off  period=1  inputsTable={'boundInpExpr'=>['','','','',''],'inputs'=>['RST','FIFO_Count0','FIFO_Count1','N_FB_TX_frame','N_FB_TX_frameTot']}  outputsTable={'outputs'=>['sel'],'suppressOut'=>['off']}  dbl_ovrd=off  enable_stdout=off  enable_debug=off  suppress_output=1  defparams={}  hide_port_list={}  block_type=mcode
      settings: block_version=10.1.3
  Up Sample : xbsIndex_r4/Up Sample  sample_ratio=N1_CIC_PRESET1  copy_samples=off  dbl_ovrd=off  block_type=usamp
      settings: infoedit="Up samples input data.  Inserted values  can be zeros or copies of the most recent input sample.<P><P>Hardware notes: No hardware is needed if inserted values are copies of the input sample; otherwise, a mux and single bit flip-flop are used."  block_version=10.1.3
  Up Sample1 : xbsIndex_r4/Up Sample  sample_ratio=N1_CIC_PRESET1  copy_samples=off  dbl_ovrd=off  block_type=usamp
      settings: infoedit="Up samples input data.  Inserted values  can be zeros or copies of the most recent input sample.<P><P>Hardware notes: No hardware is needed if inserted values are copies of the input sample; otherwise, a mux and single bit flip-flop are used."  block_version=10.1.3
  Write from FIFO (after RCH) to DAC : xbsIndex_r4/Relational  mode=a=b  en=off  latency=1  dbl_ovrd=off  block_type=relational
      settings: block_version=10.1.3
  Write from FIFO (before RCH) to RCH (befor SMQ) : xbsIndex_r4/Relational  mode=a=b  en=off  latency=1  dbl_ovrd=off  block_type=relational
      settings: block_version=10.1.3
  XOR : xbsIndex_r4/Logical  logical_function=XOR  inputs=2  en=off  latency=0  precision=Full  arith_type=Unsigned  n_bits=16  bin_pt=0  align_bp=on  dbl_ovrd=off  block_type=logical
  wires:
  Constant3/1 -> Custom register1/1
  Bit packer 1/1 -> Scope2/1, RTDEx to RCH Part/1(RTDEx_data_in)
  Sine Wave1/1 -> Bit packer 1/1, Bit packer 1/2, Scope2/2
  RTDEx to RCH Part/4(FIFO_dcount) -> [FIFO_RCH_dcount]
  RTDEx to RCH Part/1(RCH_data) -> [FIFO_RCH_InData]
  RTDEx to RCH Part/2(RCH_frame) -> [FIFO_RCH_InFrame]
  RTDEx to RCH Part/3(RCH_dvalid) -> [FIFO_RCH_InDValid]
  [FIFO_RCH_InData] -> FIFO0/1, FIFO1/1
  [FIFO_RCH_InFrame] -> Expression/1
  Custom register1/1 -> Relational/1, Relational2/1
  [RST] -> RTDEx to RCH Part/2(FIFO_rst)
  Constant1/1 -> Read from RTDEx (Host) to FIFO (befor RCH)/2
  Constant2/1 -> Write from FIFO (before RCH) to RCH (befor SMQ)/2
  Constant/1 -> Relational/2
  Relational/1 -> [RST]
  Read from RTDEx (Host) to FIFO (befor RCH)/1 -> [Re_RTDEx_to_FIFO]
  [Re_RTDEx_to_FIFO] -> RTDEx to RCH Part/3(Re_from_RTDEx_to_FIFO)
  Slice/1 -> Reinterpret/1
  Slice1/1 -> Reinterpret1/1
  Reinterpret/1 -> Mux3/3, Down Sample/1
  Reinterpret1/1 -> Down Sample1/1, Mux4/3
  Write from FIFO (after RCH) to DAC/1 -> [Write_FIFO_to_DAC]
  Constant4/1 -> Write from FIFO (after RCH) to DAC/2
  FIFO0/2 -> [F_Empty0]
  Expression1/1 -> FIFO0/3, [re0]
  Inverter3/1 -> Expression1/2
  Custom register2/1 -> Display2/1
  Status register/1 -> Display3/1
  [FIFO_RCH_dcount] -> MCode/2
  Constant12/1 -> MCode/3
  [RST] -> MCode/1
  [BufferSwap] -> MCode/4
  Constant13/1 -> [N_FB_TX_FrmLen]
  MCode/1 -> Read from RTDEx (Host) to FIFO (befor RCH)/1, Write from FIFO (before RCH) to RCH (befor SMQ)/1, Write from FIFO (after RCH) to DAC/1, Status register/1
  FIFO1/5 -> Custom register4/1, [I_Count1]
  Inverter2/1 -> Expression2/2
  FIFO1/2 -> [F_Empty1]
  Expression2/1 -> [re1], FIFO1/3
  Switch FIFOs/1 -> Convert/1
  Inverter7/1 -> [F_Sel1]
  Convert/1 -> Inverter7/1, [F_Sel0]
  [N_FB_TX_FrmLen] -> "Stop Writing if complete frame (tests for len-1, then latency 1)"/2
  Expression3/1 -> [we0], FIFO0/2
  Expression/1 -> Expression3/1, Expression4/1
  Expression4/1 -> [we1], FIFO1/2
  "Stop Writing if complete frame (tests for len-1, then latency 1)"/1 -> Inverter4/1
  Custom register4/1 -> Display5/1
  Stop Writing if complete frame1/1 -> Inverter5/1
  [F_Sel0] -> Mux1/1
  [F_Sel0] -> Expression2/1
  [F_Sel1] -> Expression4/3
  [F_Sel1] -> Expression1/1
  [N_FB_TX_FrmLen] -> Stop Writing if complete frame1/2
  [RST] -> Counter/1
  Register/1 -> XOR/2
  XOR/1 -> Counter/2, [BufferSwap]
  Counter/1 -> Custom register6/1
  [F_Sel0] -> XOR/1, Register/1
  [I_Count0] -> Switch FIFOs/2
  [I_Count0] -> "Stop Writing if complete frame (tests for len-1, then latency 1)"/1
  Inverter4/1 -> [isfull_Count0]
  [isfull_Count0] -> Expression3/2
  [I_Count1] -> Stop Writing if complete frame1/1
  [I_Count1] -> Switch FIFOs/3
  [RST] -> Switch FIFOs/1
  Inverter5/1 -> [isfull_Count1]
  [RST] -> FIFO1/4
  [RST] -> FIFO0/4
  [F_Empty0] -> Inverter3/1
  [F_Empty1] -> Inverter2/1
  FIFO0/1 -> [I_FifoOut0]
  FIFO1/1 -> [I_FifoOut1]
  [I_FifoOut0] -> Mux1/2
  [I_FifoOut1] -> Mux1/3
  [F_Sel0] -> Expression3/3
  [isfull_Count1] -> Expression4/2
  FIFO0/5 -> [I_Count0], Custom register2/1
  [F_DelayFIFO] -> Expression1/3
  [F_DelayFIFO] -> Expression2/3
  Constant6/1 -> [N_FB_TX_FrmLenTot]
  [N_FB_TX_FrmLenTot] -> Switch FIFOs/5
  [N_FB_TX_FrmLen] -> Switch FIFOs/4
  8 Bit Counter/1 -> Relational1/1
  Relational1/1 -> 8 Bit Counter/1, [F_DelayFIFO]
  "DAC Upsampling (0==no,1==2x,2==3x,...) "/1 -> Slice5/1, [I_OSFactor_1]
  Write from FIFO (before RCH) to RCH (befor SMQ)/1 -> [Write_FIFO_to_RCH]
  OR1/1 -> RTDEx to RCH Part/4(We_from_FIFO_to_RCH)
  [Flush_FIFO] -> OR1/1
  [Write_FIFO_to_RCH] -> OR1/2
  CIC Filter/1(Out1) -> Slice2/1
  CIC Filter1/1(Out1) -> Slice4/1
  Slice2/1 -> Reinterpret2/1
  Slice4/1 -> Reinterpret3/1
  Mux1/1 -> IQ demux/1
  Down Sample/1 -> CIC Filter/1(In1), Up Sample1/1
  Down Sample1/1 -> CIC Filter1/1(In1), Up Sample/1
  Constant5/1 -> Relational2/2
  Relational2/1 -> [Flush_FIFO]
  Constant8/1 -> Custom register5/1
  Custom register5/1 -> Slice3/1
  Mux5/1 -> Mux3/1, Mux4/1, Mux7/1
  Slice3/1 -> [Interpolate_Mode]
  Concat1/1 -> Status register1/1
  Constant7/1 -> Concat1/5
  Model Identification/1 -> Concat1/4
  Model Revision/1 -> Concat1/3
  Model specific parameters/1 -> Concat1/2
  Magic binary 0110/1 -> Concat1/1
  Reinterpret2/1 -> Mux3/4
  Reinterpret3/1 -> Mux4/4
  Mux3/1 -> DAC/1, DAC/3
  Mux4/1 -> DAC/2, DAC/4
  IQ demux/1 -> Slice/1
  IQ demux/2 -> Slice1/1
  [FIFO_RCH_InDValid] -> Expression/2
  Constant9/1 -> "DAC Upsampling (0==no,1==2x,2==3x,...) "/1
  Slice5/1 -> Relational1/2
  Up Sample/1 -> Mux4/2
  Up Sample1/1 -> Mux3/2
  [I_OSFactor_1] -> "If not current oversampling factor is not fixed CIC oversampling, ignore Interpolate mode and do  Sample/Hold"/1
  CIC Fixed Oversampling Factor - 1/1 -> "If not current oversampling factor is not fixed CIC oversampling, ignore Interpolate mode and do  Sample/Hold"/2
  "If not current oversampling factor is not fixed CIC oversampling, ignore Interpolate mode and do  Sample/Hold"/1 -> Mux5/1
  [Interpolate_Mode] -> Mux5/3
  Sample/Hold/1 -> Mux5/2
  Mux6/1 -> Inverter6/1
  [F_Sel0] -> Mux6/1
  [F_Empty0] -> Mux6/2
  [F_Empty1] -> Mux6/3
  Inverter6/1 -> Mux7/2, Mux7/3, Delay1/1
  Delay1/1 -> Mux7/4
  Mux7/1 -> DAC/5
